simulink model "RoboBoatVU_2014_Dionysus"  (R2014a)
settings: Solver=FixedStepDiscrete  StartTime=0.0  StopTime=inf  FixedStep=.1  RelTol=1e-3
undefined symbols (not defined in the file): Com1, Com2, Com3, Com4, DiscIntNeverNeededParam, RGB24, standard
libraries: visiontextngfix x66, simulink x53, xpcseriallib x15, dspmtrx3 x14, slrtlib x3, speedgoatlib_IO102 x3, visionstatistics x2, dspstat3 x2, dspindex x2, xpcvideousblib x2, xpcvideoutillib x2, speedgoatlib x1
(part 1 of 7)
settings Model: BufferReuse=off  Creator=wildcat  LastModifiedBy=wildcat
settings SolverCC: EnableConcurrentExecution=on
settings DataIOCC: SignalLoggingSaveFormat=ModelDataLogs
settings OptimizationCC: BlockReduction=off  OptimizeBlockIOStorage=off  BufferReuse=off  GlobalBufferReuse=off  ExpressionFolding=off  LocalBlockOutputs=off
settings DebuggingCC: UnderspecifiedInitializationDetection=Classic  StateNameClashWarn=warning
settings HardwareCC: ProdIntDivRoundTo=Zero  ProdEndianess=LittleEndian  ProdHWDeviceType=Generic->32-bit x86 compatible
settings RTWCC: SystemTargetFile=slrt.tlc  TemplateMakefile=slrt_default_tmf  Description=Simulink Real-Time  ProcessScript=slrt_make_rtw_hook  RTWCompilerOptimization=On
settings SimulinkRealTimeCC: GeneratePreprocessorConditionals=Disable all  EnableShiftOperators=on

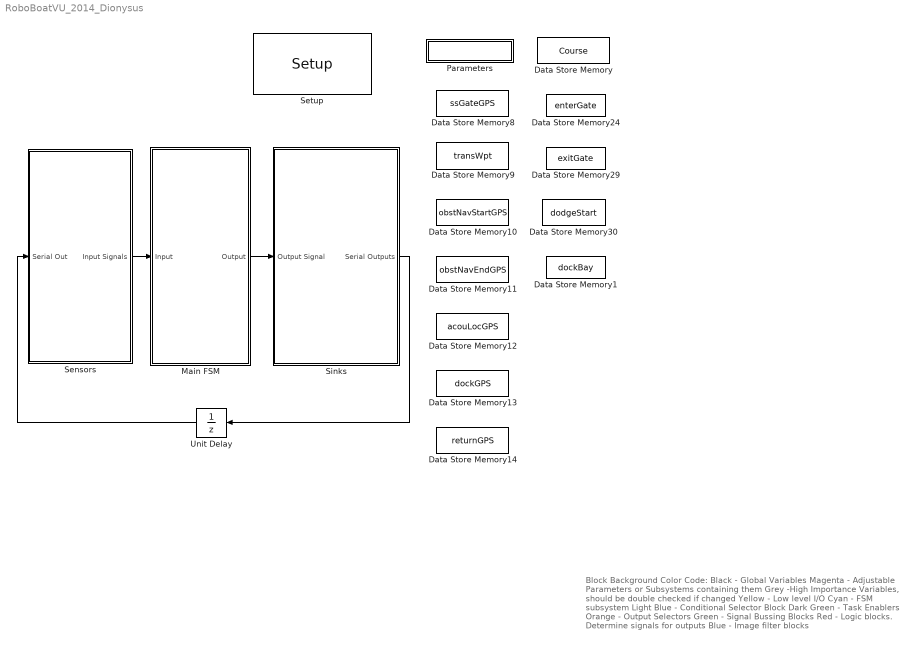
== system RoboBoatVU_2014_Dionysus ==
  note: Block Background Color Code:
      | Black - Global Variables
      | Magenta - Adjustable Parameters or Subsystems containing them
      | Grey -High Importance Variables, should be double checked if changed
      | Yellow - Low level I/O
      | Cyan - FSM subsystem
      | Light Blue - Conditional Selector Block
      | Dark Green - Task Enablers
      | Orange - Output Selectors
      | Green - Signal Bussing Blocks
      | Red - Logic blocks. Determine signals for outputs
      | Blue - Image filter blocks
  Data Store Memory : DataStoreMemory  DataStoreName=Course  ReadBeforeWriteMsg=warning  WriteAfterWriteMsg=warning  WriteAfterReadMsg=warning
  Data Store Memory1 : DataStoreMemory  DataStoreName=dockBay  ReadBeforeWriteMsg=warning  WriteAfterWriteMsg=warning  WriteAfterReadMsg=warning
  Data Store Memory10 : DataStoreMemory  DataStoreName=obstNavStartGPS  ReadBeforeWriteMsg=warning  WriteAfterWriteMsg=warning  WriteAfterReadMsg=warning  InitialValue=zeros(1,2)
  Data Store Memory11 : DataStoreMemory  DataStoreName=obstNavEndGPS  ReadBeforeWriteMsg=warning  WriteAfterWriteMsg=warning  WriteAfterReadMsg=warning  InitialValue=zeros(1,2)
  Data Store Memory12 : DataStoreMemory  DataStoreName=acouLocGPS  ReadBeforeWriteMsg=warning  WriteAfterWriteMsg=warning  WriteAfterReadMsg=warning  InitialValue=zeros(1,2)
  Data Store Memory13 : DataStoreMemory  DataStoreName=dockGPS  ReadBeforeWriteMsg=warning  WriteAfterWriteMsg=warning  WriteAfterReadMsg=warning  InitialValue=zeros(1,2)
  Data Store Memory14 : DataStoreMemory  DataStoreName=returnGPS  ReadBeforeWriteMsg=warning  WriteAfterWriteMsg=warning  WriteAfterReadMsg=warning  InitialValue=zeros(1,2)
  Data Store Memory24 : DataStoreMemory  DataStoreName=enterGate  ReadBeforeWriteMsg=warning  WriteAfterWriteMsg=warning  WriteAfterReadMsg=warning
  Data Store Memory29 : DataStoreMemory  DataStoreName=exitGate  ReadBeforeWriteMsg=warning  WriteAfterWriteMsg=warning  WriteAfterReadMsg=warning
  Data Store Memory30 : DataStoreMemory  DataStoreName=dodgeStart  ReadBeforeWriteMsg=warning  WriteAfterWriteMsg=warning  WriteAfterReadMsg=warning
  Data Store Memory8 : DataStoreMemory  DataStoreName=ssGateGPS  ReadBeforeWriteMsg=warning  WriteAfterWriteMsg=warning  WriteAfterReadMsg=warning  InitialValue=zeros(1,2)
  Data Store Memory9 : DataStoreMemory  DataStoreName=transWpt  ReadBeforeWriteMsg=warning  WriteAfterWriteMsg=warning  WriteAfterReadMsg=warning  InitialValue=zeros(1,2)
  Main FSM : Subsystem
  Parameters : Subsystem
  Sensors : Subsystem
  Setup : speedgoatlib_IO102/Setup  group=Digital output setup  id=1  range=+-5V  cal=off  pciSlot=-1  adChannelMode=Multiple-channel (enter number of channels below)  adChannel=16  adCoupling=Differential  daChannel=[1,2,3,4]  daReset=[1]  daInitValue=[0]  diChannel=[1,2,3,4,5,6,7,8]  doChannel=[1,2,3,4,5,6,7,8]  doReset=[1]  doInitValue=[0]
  Sinks : Subsystem
  Unit Delay : UnitDelay  SampleTime=-1
  wires:
  Main FSM/1(Output) -> Sinks/1(Output Signal)
  Sensors/1(Input Signals) -> Main FSM/1(Input)
  Sinks/1(Serial Outputs) -> Unit Delay/1
  Unit Delay/1 -> Sensors/1(Serial Out)

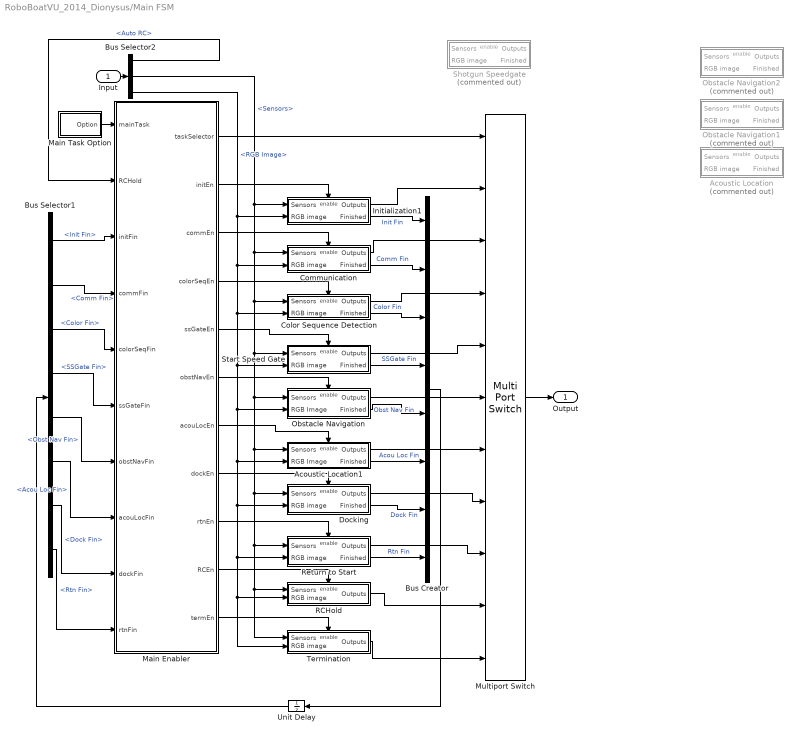
== system RoboBoatVU_2014_Dionysus/Main FSM ==
  Input : Inport
  Acoustic Location : Subsystem  Commented=on  TreatAsAtomicUnit=on
  Acoustic Location1 : Subsystem  TreatAsAtomicUnit=on
  Bus Creator : BusCreator  Inputs=8
  Bus Selector1 : BusSelector  OutputSignals=Init Fin,Comm Fin,Color Fin,SSGate Fin,Obst Nav Fin,Acou Loc Fin,Dock Fin,Rtn Fin
  Bus Selector2 : BusSelector  OutputSignals=Sensors.Digital In.Auto RC,Sensors,RGB Image
  Color Sequence Detection : Subsystem  TreatAsAtomicUnit=on
  Communication : Subsystem
  Docking : Subsystem  TreatAsAtomicUnit=on
  Initialization1 : Subsystem
  Main Enabler : MATLAB Function  TreatAsAtomicUnit=on
  Main Task Option : Subsystem
  Multiport Switch : MultiPortSwitch  Inputs=10
  Obstacle Navigation : Subsystem  TreatAsAtomicUnit=on
  Obstacle Navigation1 : Subsystem  Commented=on  TreatAsAtomicUnit=on
  Obstacle Navigation2 : Subsystem  Commented=on  TreatAsAtomicUnit=on
  RCHold : Subsystem
  Return to Start : Subsystem  TreatAsAtomicUnit=on
  Shotgun Speedgate : Subsystem  Commented=on  TreatAsAtomicUnit=on
  Start Speed Gate : Subsystem  TreatAsAtomicUnit=on
  Termination : Subsystem  TreatAsAtomicUnit=on
  Unit Delay : UnitDelay  SampleTime=-1
  Output : Outport
  wires:
  Bus Creator/1 -> Unit Delay/1
  Initialization1/1(Outputs) -> Multiport Switch/2
  Multiport Switch/1 -> Output/1
  Main Task Option/1(Option) -> Main Enabler/1(mainTask)
  Main Enabler/1(taskSelector) -> Multiport Switch/1
  Initialization1/2(Finished) -> Bus Creator/1  "Init Fin"
  Unit Delay/1 -> Bus Selector1/1
  Input/1 -> Bus Selector2/1
  Bus Selector2/1 -> Main Enabler/2(RCHold)  "<Auto RC>"
  Main Enabler/2(initEn) -> Initialization1/Enable
  Termination/1(Outputs) -> Multiport Switch/11
  RCHold/1(Outputs) -> Multiport Switch/10
  Main Enabler/10(RCEn) -> RCHold/Enable
  Main Enabler/11(termEn) -> Termination/Enable
  Bus Selector2/2 -> Communication/1(Sensors), Color Sequence Detection/1(Sensors), Start Speed Gate/1(Sensors), Obstacle Navigation/1(Sensors), Docking/1(Sensors), Return to Start/1(Sensors), RCHold/1(Sensors), Termination/1(Sensors), Acoustic Location1/1(Sensors), Initialization1/1(Sensors)  "<Sensors>"
  Bus Selector2/3 -> Communication/2(RGB image), Color Sequence Detection/2(RGB image), Start Speed Gate/2(RGB image), Obstacle Navigation/2(RGB Image), Docking/2(RGB image), Return to Start/2(RGB image), Termination/2(RGB image), RCHold/2(RGB image), Acoustic Location1/2(RGB Image), Initialization1/2(RGB image)  "<RGB Image>"
  Color Sequence Detection/2(Finished) -> Bus Creator/3  "Color Fin"
  Start Speed Gate/2(Finished) -> Bus Creator/4  "SSGate Fin"
  Obstacle Navigation/2(Finished) -> Bus Creator/5  "Obst Nav Fin"
  Acoustic Location1/2(Finished) -> Bus Creator/6  "Acou Loc Fin"
  Docking/2(Finished) -> Bus Creator/7  "Dock Fin"
  Return to Start/2(Finished) -> Bus Creator/8  "Rtn Fin"
  Return to Start/1(Outputs) -> Multiport Switch/9
  Docking/1(Outputs) -> Multiport Switch/8
  Acoustic Location1/1(Outputs) -> Multiport Switch/7
  Obstacle Navigation/1(Outputs) -> Multiport Switch/6
  Start Speed Gate/1(Outputs) -> Multiport Switch/5
  Color Sequence Detection/1(Outputs) -> Multiport Switch/4
  Main Enabler/4(colorSeqEn) -> Color Sequence Detection/Enable
  Main Enabler/5(ssGateEn) -> Start Speed Gate/Enable
  Main Enabler/6(obstNavEn) -> Obstacle Navigation/Enable
  Main Enabler/7(acouLocEn) -> Acoustic Location1/Enable
  Main Enabler/8(dockEn) -> Docking/Enable
  Main Enabler/9(rtnEn) -> Return to Start/Enable
  Bus Selector1/7 -> Main Enabler/9(dockFin)  "<Dock Fin>"
  Bus Selector1/1 -> Main Enabler/3(initFin)  "<Init Fin>"
  Bus Selector1/5 -> Main Enabler/7(obstNavFin)  "<Obst Nav Fin>"
  Bus Selector1/6 -> Main Enabler/8(acouLocFin)  "<Acou Loc Fin>"
  Bus Selector1/3 -> Main Enabler/5(colorSeqFin)  "<Color Fin>"
  Bus Selector1/4 -> Main Enabler/6(ssGateFin)  "<SSGate Fin>"
  Bus Selector1/8 -> Main Enabler/10(rtnFin)  "<Rtn Fin>"
  Main Enabler/3(commEn) -> Communication/Enable
  Communication/2(Finished) -> Bus Creator/2  "Comm Fin"
  Communication/1(Outputs) -> Multiport Switch/3
  Bus Selector1/2 -> Main Enabler/4(commFin)  "<Comm Fin>"

== system RoboBoatVU_2014_Dionysus/Parameters ==
  note: Course options are:
      | A, B and
      | otherwise (for testing,
      |  must be one character)
  CourseName : Constant  Value=uint8('B')  VectorParams1D=off
  GPS Points : Subsystem
  Write : DataStoreWrite  DataStoreName=Course
  wires:
  CourseName/1 -> Write/1

== system RoboBoatVU_2014_Dionysus/Sensors ==
  Serial Out : Inport
  Bus Creator : BusCreator  Inputs=2
  Bus Creator1 : BusCreator  Inputs=2
  Digital In : Subsystem
  Serial In : Subsystem
  Video In : Subsystem
  Input Signals : Outport
  wires:
  Serial In/1(Serial In) -> Bus Creator/1
  Digital In/1(Digital In) -> Bus Creator/2
  Video In/1(RGB image) -> Bus Creator1/2
  Bus Creator/1 -> Bus Creator1/1  "Sensors"
  Bus Creator1/1 -> Input Signals/1
  Serial Out/1 -> Serial In/1(Serial Out)

== system RoboBoatVU_2014_Dionysus/Sinks ==
  Output Signal : Inport
  Bus Selector : BusSelector  OutputSignals=Sensors.Serial In.Compass.Heading,Outputs.Control Signals,Outputs.Annotated Image,Outputs.Serial Outputs
  Image Transmission : Subsystem
  actuators : Subsystem
  data log : Subsystem  Commented=on
  Serial Outputs : Outport
  wires:
  Bus Selector/2 -> actuators/2(Control Signals)  "<Control Signals>"
  Bus Selector/3 -> Image Transmission/1(RGB Image)  "<Annotated Image>"
  Bus Selector/1 -> actuators/1(Compass Heading)  "<Heading>"
  Output Signal/1 -> data log/1(Output signal), Bus Selector/1
  Bus Selector/4 -> Serial Outputs/1  "<Serial Outputs>"

== system RoboBoatVU_2014_Dionysus/Main FSM/Acoustic Location ==
  note: Acoustic Location
  Sensors : Inport
  RGB image : Inport  Port=2
  Enable : EnablePort  ShowOutputPort=on
  Annotate Task : visiontextngfix/Insert Text  inputType=Obsolete  theText='Acoustic Location...'  getTextLocFrom=Specify via dialog  textLoc=[10 10]  getTextColorFrom=Specify via dialog  textColor=[0 0 255]  getTextIntensityFrom=Specify via dialog  textIntensity=0  getTextOpacityFrom=Specify via dialog  textOpacity=1.0  dummyVar2=0  dummyVar3=0  dummyVar4=0  imagePorts=One multidimensional signal  isInputTransposed=off  fontFace=LucidaSansRegular  dummyVar1=0  blockFontSize=12  antiAliased=on
  Bus Selector : BusSelector  OutputSignals=Serial In.Compass.Heading
  Compare To Constant : simulink/Logic and Bit Operations/Compare To Constant  relop=>=  const=10  OutDataTypeStr=boolean
  Constant : Constant  Value=0
  Data Type Conversion : DataTypeConversion  OutDataTypeStr=double
  Discrete-Time Integrator : DiscreteIntegrator  SampleTime=0.1  ICPrevOutput=DiscIntNeverNeededParam  ICPrevScaledInput=DiscIntNeverNeededParam
  Output Heirarchy : Subsystem
  Outputs : Outport
  Finished : Outport  Port=2
  wires:
  Sensors/1 -> Output Heirarchy/3(Sensors), Bus Selector/1  "Sensors"
  Bus Selector/1 -> Output Heirarchy/2(Desired Heading)  "<Heading>"
  RGB image/1 -> Annotate Task/1
  Annotate Task/1 -> Output Heirarchy/1(Annotated Image)
  Output Heirarchy/1(Outputs) -> Outputs/1
  Compare To Constant/1 -> Data Type Conversion/1
  Enable/1 -> Discrete-Time Integrator/1
  Discrete-Time Integrator/1 -> Compare To Constant/1
  Constant/1 -> Output Heirarchy/4(Request Number)
  Data Type Conversion/1 -> Finished/1

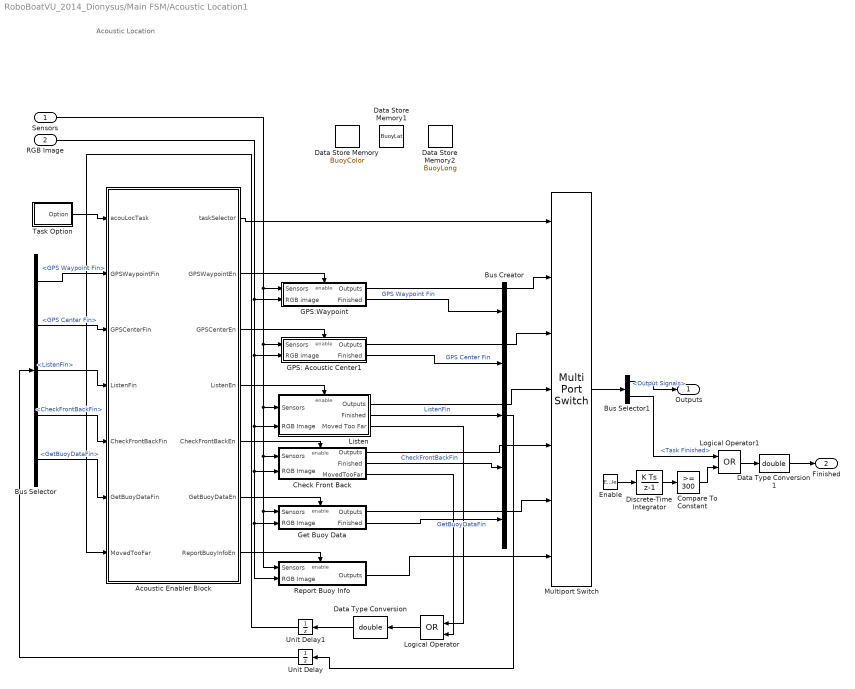
== system RoboBoatVU_2014_Dionysus/Main FSM/Acoustic Location1 ==
  note: Acoustic Location
  Sensors : Inport
  RGB Image : Inport  Port=2
  Enable : EnablePort  ShowOutputPort=on
  Acoustic Enabler Block : MATLAB Function  TreatAsAtomicUnit=on
  Bus Creator : BusCreator  Inputs=5
  Bus Selector : BusSelector  OutputSignals=GPS Waypoint Fin,GPS Center Fin,ListenFin,CheckFrontBackFin,GetBuoyDataFin
  Bus Selector1 : BusSelector  OutputSignals=Output Signals,Task Finished
  Check Front Back : Subsystem  TreatAsAtomicUnit=on
  Compare To Constant : simulink/Logic and Bit Operations/Compare To Constant  relop=>=  const=300  OutDataTypeStr=boolean
  Data Store Memory : DataStoreMemory  DataStoreName=BuoyColor  ReadBeforeWriteMsg=warning  WriteAfterWriteMsg=warning  WriteAfterReadMsg=warning
  Data Store Memory1 : DataStoreMemory  DataStoreName=BuoyLat  ReadBeforeWriteMsg=warning  WriteAfterWriteMsg=warning  WriteAfterReadMsg=warning
  Data Store Memory2 : DataStoreMemory  DataStoreName=BuoyLong  ReadBeforeWriteMsg=warning  WriteAfterWriteMsg=warning  WriteAfterReadMsg=warning
  Data Type Conversion : DataTypeConversion  OutDataTypeStr=double
  Data Type Conversion1 : DataTypeConversion  OutDataTypeStr=double
  Discrete-Time Integrator : DiscreteIntegrator  SampleTime=0.1  ICPrevOutput=DiscIntNeverNeededParam  ICPrevScaledInput=DiscIntNeverNeededParam
  GPS: Acoustic Center1 : Subsystem  TreatAsAtomicUnit=on
  GPS:Waypoint : Subsystem  TreatAsAtomicUnit=on
  Get Buoy Data : Subsystem  TreatAsAtomicUnit=on
  Listen : Subsystem  TreatAsAtomicUnit=on
  Logical Operator : Logic  Operator=OR  IconShape=distinctive  AllPortsSameDT=off  OutDataTypeStr=boolean
  Logical Operator1 : Logic  Operator=OR  AllPortsSameDT=off  OutDataTypeStr=boolean
  Multiport Switch : MultiPortSwitch  Inputs=6
  Report Buoy Info : Subsystem  TreatAsAtomicUnit=on
  Task Option : Subsystem
  Unit Delay : UnitDelay  SampleTime=-1
  Unit Delay1 : UnitDelay  SampleTime=-1
  Outputs : Outport
  Finished : Outport  Port=2
  wires:
  Sensors/1 -> GPS:Waypoint/1(Sensors), GPS: Acoustic Center1/1(Sensors), Report Buoy Info/1(Sensors), Get Buoy Data/1(Sensors), Check Front Back/1(Sensors), Listen/1(Sensors)
  RGB Image/1 -> GPS:Waypoint/2(RGB image), GPS: Acoustic Center1/2(RGB image), Report Buoy Info/2(RGB Image), Get Buoy Data/2(RGB Image), Check Front Back/2(RGB Image), Listen/2(RGB Image)
  Acoustic Enabler Block/1(taskSelector) -> Multiport Switch/1
  Acoustic Enabler Block/3(GPSCenterEn) -> GPS: Acoustic Center1/Enable
  Acoustic Enabler Block/4(ListenEn) -> Listen/Enable
  Acoustic Enabler Block/5(CheckFrontBackEn) -> Check Front Back/Enable
  Acoustic Enabler Block/7(ReportBuoyInfoEn) -> Report Buoy Info/Enable
  Listen/1(Outputs) -> Multiport Switch/4
  Check Front Back/1(Outputs) -> Multiport Switch/5
  Report Buoy Info/1(Outputs) -> Multiport Switch/7
  Listen/2(Finished) -> Bus Creator/3  "ListenFin"
  Check Front Back/2(Finished) -> Bus Creator/4  "CheckFrontBackFin"
  Unit Delay/1 -> Bus Selector/1
  Bus Selector/2 -> Acoustic Enabler Block/3(GPSCenterFin)  "<GPS Center Fin>"
  Multiport Switch/1 -> Bus Selector1/1
  GPS: Acoustic Center1/1(Outputs) -> Multiport Switch/3
  GPS: Acoustic Center1/2(Finished) -> Bus Creator/2  "GPS Center Fin"
  Bus Creator/1 -> Unit Delay/1
  Get Buoy Data/1(Outputs) -> Multiport Switch/6
  Get Buoy Data/2(Finished) -> Bus Creator/5  "GetBuoyDataFin"
  Bus Selector/5 -> Acoustic Enabler Block/6(GetBuoyDataFin)  "<GetBuoyDataFin>"
  Bus Selector/3 -> Acoustic Enabler Block/4(ListenFin)  "<ListenFin>"
  Bus Selector/4 -> Acoustic Enabler Block/5(CheckFrontBackFin)  "<CheckFrontBackFin>"
  Acoustic Enabler Block/6(GetBuoyDataEn) -> Get Buoy Data/Enable
  Task Option/1(Option) -> Acoustic Enabler Block/1(acouLocTask)
  Listen/3(Moved Too Far) -> Logical Operator/1
  Unit Delay1/1 -> Acoustic Enabler Block/7(MovedTooFar)
  Check Front Back/3(MovedTooFar) -> Logical Operator/2
  Logical Operator/1 -> Data Type Conversion/1
  Data Type Conversion/1 -> Unit Delay1/1
  Acoustic Enabler Block/2(GPSWaypointEn) -> GPS:Waypoint/Enable
  GPS:Waypoint/1(Outputs) -> Multiport Switch/2
  GPS:Waypoint/2(Finished) -> Bus Creator/1  "GPS Waypoint Fin"
  Bus Selector1/1 -> Outputs/1  "<Output Signals>"
  Bus Selector/1 -> Acoustic Enabler Block/2(GPSWaypointFin)  "<GPS Waypoint Fin>"
  Enable/1 -> Discrete-Time Integrator/1
  Discrete-Time Integrator/1 -> Compare To Constant/1
  Logical Operator1/1 -> Data Type Conversion1/1
  Bus Selector1/2 -> Logical Operator1/1  "<Task Finished>"
  Compare To Constant/1 -> Logical Operator1/2
  Data Type Conversion1/1 -> Finished/1

== system RoboBoatVU_2014_Dionysus/Main FSM/Color Sequence Detection ==
  note: Color Sequence Detection
  Sensors : Inport
  RGB image : Inport  Port=2
  Enable : EnablePort
  Main Enabler : MATLAB Function  TreatAsAtomicUnit=on
  Main Selector : MultiPortSwitch  Inputs=2
  Output Reassign : Subsystem
  Report : Subsystem  TreatAsAtomicUnit=on
  Request : Subsystem  TreatAsAtomicUnit=on
  Unit Delay : UnitDelay  SampleTime=-1
  Outputs : Outport
  Finished : Outport  Port=2
  wires:
  Main Enabler/2(RequestEn) -> Request/Enable
  Sensors/1 -> Request/1(Sensors), Report/1(Sensors)
  RGB image/1 -> Request/2(RGB image), Report/2(RGB image)
  Request/1(Outputs) -> Main Selector/2
  Report/1(Outputs) -> Main Selector/3
  Request/2(Finished) -> Unit Delay/1
  Unit Delay/1 -> Main Enabler/1(RequestFin)
  Main Enabler/1(taskSelector) -> Main Selector/1
  Main Enabler/3(ReportEn) -> Report/Enable
  Main Selector/1 -> Output Reassign/1(Outputs in)
  Output Reassign/1(Outputs) -> Outputs/1
  Output Reassign/2(Finished) -> Finished/1

== system RoboBoatVU_2014_Dionysus/Main FSM/Communication ==
  Sensors : Inport
  RGB image : Inport  Port=2
  Enable : EnablePort
  Docking Bay Comm : Subsystem  TreatAsAtomicUnit=on
  Main Enabler : MATLAB Function  TreatAsAtomicUnit=on
  Main Selector : MultiPortSwitch  Inputs=2
  Obst Gate Comm : Subsystem  TreatAsAtomicUnit=on
  Output Reassign : Subsystem
  Unit Delay : UnitDelay  SampleTime=-1
  Outputs : Outport
  Finished : Outport  Port=2
  wires:
  Main Enabler/2(ObstCommEn) -> Obst Gate Comm/Enable
  Sensors/1 -> Docking Bay Comm/1(Sensors), Obst Gate Comm/1(Sensors)
  RGB image/1 -> Docking Bay Comm/2(RGB image), Obst Gate Comm/2(RGB image)
  Obst Gate Comm/1(Outputs) -> Main Selector/2
  Docking Bay Comm/1(Outputs) -> Main Selector/3
  Obst Gate Comm/2(Finished) -> Unit Delay/1
  Unit Delay/1 -> Main Enabler/1(ObstCommFin)
  Main Enabler/1(taskSelector) -> Main Selector/1
  Main Enabler/3(DockingCommEn) -> Docking Bay Comm/Enable
  Main Selector/1 -> Output Reassign/1(Outputs in)
  Output Reassign/1(Outputs) -> Outputs/1
  Output Reassign/2(Finished) -> Finished/1

== system RoboBoatVU_2014_Dionysus/Main FSM/Docking ==
  note: Docking
  Sensors : Inport
  RGB image : Inport  Port=2
  Enable : EnablePort  ShowOutputPort=on
  Annotate Task : visiontextngfix/Insert Text  inputType=Obsolete  theText='Docking...'  getTextLocFrom=Specify via dialog  textLoc=[10 10]  getTextColorFrom=Specify via dialog  textColor=[0 0 255]  getTextIntensityFrom=Specify via dialog  textIntensity=0  getTextOpacityFrom=Specify via dialog  textOpacity=1.0  dummyVar2=0  dummyVar3=0  dummyVar4=0  imagePorts=One multidimensional signal  isInputTransposed=off  fontFace=LucidaSansRegular  dummyVar1=0  blockFontSize=12  antiAliased=on
  Annotate Task1 : visiontextngfix/Insert Text  inputType=Obsolete  theText='Symbol: %f'  getTextLocFrom=Specify via dialog  textLoc=[10 20]  getTextColorFrom=Specify via dialog  textColor=[0 0 255]  getTextIntensityFrom=Specify via dialog  textIntensity=0  getTextOpacityFrom=Specify via dialog  textOpacity=1.0  dummyVar2=0  dummyVar3=0  dummyVar4=0  imagePorts=One multidimensional signal  isInputTransposed=off  fontFace=LucidaSansRegular  dummyVar1=0  blockFontSize=12  antiAliased=on
  Bus Selector : BusSelector  OutputSignals=Serial In.Comms.Dat1,Serial In.Compass.Heading
  Compare To Constant : simulink/Logic and Bit Operations/Compare To Constant  relop=>=  const=5  OutDataTypeStr=boolean
  Constant : Constant  Value=2
  Data Type Conversion : DataTypeConversion  OutDataTypeStr=double
  Discrete-Time Integrator : DiscreteIntegrator  SampleTime=0.1  ICPrevOutput=DiscIntNeverNeededParam  ICPrevScaledInput=DiscIntNeverNeededParam
  Output Heirarchy : Subsystem
  Outputs : Outport
  Finished : Outport  Port=2
  wires:
  Sensors/1 -> Bus Selector/1, Output Heirarchy/3(Sensors)  "Sensors"
  Bus Selector/2 -> Output Heirarchy/2(Desired Heading)  "<Heading>"
  RGB image/1 -> Annotate Task/1
  Output Heirarchy/1(Outputs) -> Outputs/1
  Compare To Constant/1 -> Data Type Conversion/1
  Enable/1 -> Discrete-Time Integrator/1
  Discrete-Time Integrator/1 -> Compare To Constant/1
  Constant/1 -> Output Heirarchy/4(Request Number)
  Annotate Task/1 -> Annotate Task1/1
  Bus Selector/1 -> Annotate Task1/2  "<Dat1>"
  Annotate Task1/1 -> Output Heirarchy/1(Annotated Image)
  Data Type Conversion/1 -> Finished/1

== system RoboBoatVU_2014_Dionysus/Main FSM/Initialization1 ==
  Sensors : Inport
  RGB image : Inport  Port=2
  Enable : EnablePort  ShowOutputPort=on
  Annotate Task : visiontextngfix/Insert Text  inputType=Obsolete  theText='Initializing...'  getTextLocFrom=Specify via dialog  textLoc=[10 10]  getTextColorFrom=Specify via dialog  textColor=[0 0 255]  getTextIntensityFrom=Specify via dialog  textIntensity=0  getTextOpacityFrom=Specify via dialog  textOpacity=1.0  dummyVar2=0  dummyVar3=0  dummyVar4=0  imagePorts=One multidimensional signal  isInputTransposed=off  fontFace=LucidaSansRegular  dummyVar1=0  blockFontSize=12  antiAliased=on
  Bus Selector : BusSelector  OutputSignals=Serial In.Compass.Heading
  Compare To Constant : simulink/Logic and Bit Operations/Compare To Constant  relop=>=  const=5  OutDataTypeStr=boolean
  Constant : Constant  Value=0
  Data Type Conversion : DataTypeConversion  OutDataTypeStr=double
  Discrete-Time Integrator : DiscreteIntegrator  SampleTime=0.1  ICPrevOutput=DiscIntNeverNeededParam  ICPrevScaledInput=DiscIntNeverNeededParam
  Output Heirarchy : Subsystem
  Outputs : Outport
  Finished : Outport  Port=2
  wires:
  Sensors/1 -> Bus Selector/1, Output Heirarchy/3(Sensors)  "Sensors"
  Bus Selector/1 -> Output Heirarchy/2(Desired Heading)  "<Heading>"
  RGB image/1 -> Annotate Task/1
  Annotate Task/1 -> Output Heirarchy/1(Annotated Image)
  Output Heirarchy/1(Outputs) -> Outputs/1
  Compare To Constant/1 -> Data Type Conversion/1
  Enable/1 -> Discrete-Time Integrator/1
  Discrete-Time Integrator/1 -> Compare To Constant/1
  Constant/1 -> Output Heirarchy/4(Request Number)
  Data Type Conversion/1 -> Finished/1

== system RoboBoatVU_2014_Dionysus/Main FSM/Main Task Option ==
  note: Main Task Options
  Message Composer : MATLAB Function  TreatAsAtomicUnit=on
  Test Comms Option : Constant  Value=uint8('All')  SampleTime=0.1
  Option : Outport
  wires:
  Test Comms Option/1 -> Message Composer/1(taskStrInit)
  Message Composer/1(taskStrAdj) -> Option/1

== system RoboBoatVU_2014_Dionysus/Main FSM/Obstacle Navigation ==
  note: Distance threshold changed from 2m to 3m
  note: Variables to test:
      | 1. RPM values for GPS approach and dodge subroutine
      | 2. Angle threshold for ignoring obstacle
  note: Places to change RPM value
      | Dodge/Nav Logic: 2 places
      | GPS: Bee Line/Approach/Output Heirarchy1: 1 place
  Sensors : Inport
  RGB Image : Inport  Port=2
  Enable : EnablePort  ShowOutputPort=on
  Compare To Constant1 : simulink/Logic and Bit Operations/Compare To Constant  relop=>=  const=180  OutDataTypeStr=boolean
  Data Store Read : DataStoreRead  DataStoreName=dodgeStart  SampleTime=0.1
  Data Type Conversion1 : DataTypeConversion  OutDataTypeStr=double
  Discrete-Time Integrator : DiscreteIntegrator  SampleTime=0.1  ICPrevOutput=DiscIntNeverNeededParam  ICPrevScaledInput=DiscIntNeverNeededParam
  Dodge : Subsystem  TreatAsAtomicUnit=on
  GPS: Bee Line : Subsystem  TreatAsAtomicUnit=on
  Logical Operator : Logic  Operator=OR  AllPortsSameDT=off  OutDataTypeStr=boolean
  Multiport Switch : MultiPortSwitch  Inputs=2
  Obstacle Navigation Enabler : MATLAB Function  TreatAsAtomicUnit=on
  Output Reassign : Subsystem
  Unit Delay : UnitDelay  SampleTime=-1
  Outputs : Outport
  Finished : Outport  Port=2
  wires:
  Obstacle Navigation Enabler/3(GPSEn) -> GPS: Bee Line/Enable
  Sensors/1 -> GPS: Bee Line/1(Sensors), Dodge/1(Sensors)
  RGB Image/1 -> GPS: Bee Line/2(RGB image), Dodge/2(RGB image)
  Obstacle Navigation Enabler/2(dodgeEn) -> Dodge/Enable
  Dodge/1(Outputs) -> Multiport Switch/2
  GPS: Bee Line/1(Outputs) -> Multiport Switch/3
  Obstacle Navigation Enabler/1(taskSelector) -> Multiport Switch/1
  Dodge/2(Dodge Incomplete) -> Unit Delay/1  "Dodge Incomplete"
  Data Store Read/1 -> Obstacle Navigation Enabler/2(dodgeStart)
  Unit Delay/1 -> Obstacle Navigation Enabler/1(dodgeIncomplete)
  Multiport Switch/1 -> Output Reassign/1(Outputs in)
  Output Reassign/1(Outputs) -> Outputs/1
  Output Reassign/2(Finished) -> Logical Operator/2
  Discrete-Time Integrator/1 -> Compare To Constant1/1
  Compare To Constant1/1 -> Logical Operator/1
  Enable/1 -> Discrete-Time Integrator/1
  Logical Operator/1 -> Data Type Conversion1/1
  Data Type Conversion1/1 -> Finished/1

== system RoboBoatVU_2014_Dionysus/Main FSM/Obstacle Navigation1 ==
  Sensors : Inport
  RGB image : Inport  Port=2
  Enable : EnablePort
  Bus Creator1 : BusCreator
  Bus Selector1 : BusSelector  OutputSignals=GPS Fin,Comm Fin,Enter Fin,Nav Fin
  Communication : Subsystem  TreatAsAtomicUnit=on
  Enter Gate : Subsystem  TreatAsAtomicUnit=on
  Exit Gate : Subsystem  TreatAsAtomicUnit=on
  GPS: Center : Subsystem  TreatAsAtomicUnit=on
  MATLAB Function1 : MATLAB Function  TreatAsAtomicUnit=on
  Multiport Switch1 : MultiPortSwitch  Inputs=5
  Obstacle Navigation : Subsystem  TreatAsAtomicUnit=on
  Output Reassign : Subsystem
  Task Option1 : Subsystem
  Unit Delay1 : UnitDelay  SampleTime=-1
  Outputs : Outport
  Finished : Outport  Port=2
  wires:
  Task Option1/1(Option) -> MATLAB Function1/1(taskMode)
  MATLAB Function1/2(startGPSEn) -> GPS: Center/Enable
  GPS: Center/1(Outputs) -> Multiport Switch1/2
  MATLAB Function1/1(taskSelector) -> Multiport Switch1/1
  MATLAB Function1/3(commEn) -> Communication/Enable
  MATLAB Function1/6(exitGateEn) -> Exit Gate/Enable
  MATLAB Function1/5(obstNavEn) -> Obstacle Navigation/Enable
  MATLAB Function1/4(enterGateEn) -> Enter Gate/Enable
  GPS: Center/2(Finished) -> Bus Creator1/1  "GPS Fin"
  Communication/2(Finished) -> Bus Creator1/2  "Comm Fin"
  Enter Gate/2(Finished) -> Bus Creator1/3  "Enter Fin"
  Obstacle Navigation/2(Finished) -> Bus Creator1/4  "Nav Fin"
  Obstacle Navigation/1(Outputs) -> Multiport Switch1/5
  Enter Gate/1(Outputs) -> Multiport Switch1/4
  Communication/1(Outputs) -> Multiport Switch1/3
  Bus Creator1/1 -> Unit Delay1/1
  Unit Delay1/1 -> Bus Selector1/1
  Bus Selector1/1 -> MATLAB Function1/2(startGPSFin)  "<GPS Fin>"
  Bus Selector1/2 -> MATLAB Function1/3(commFin)  "<Comm Fin>"
  Bus Selector1/3 -> MATLAB Function1/4(enterGateFin)  "<Enter Fin>"
  Bus Selector1/4 -> MATLAB Function1/5(obstNavFin)  "<Nav Fin>"
  Exit Gate/1(Outputs) -> Multiport Switch1/6
  Sensors/1 -> GPS: Center/1(Sensors), Communication/1(Sensors), Enter Gate/1(Sensors), Exit Gate/1(Sensors), Obstacle Navigation/1(Sensors)
  RGB image/1 -> GPS: Center/2(RGB image), Communication/2(RGB Image), Enter Gate/2(RGB Image), Exit Gate/2(RGB Image), Obstacle Navigation/2(RGB Image)
  Multiport Switch1/1 -> Output Reassign/1(Outputs in)
  Output Reassign/1(Outputs) -> Outputs/1
  Output Reassign/2(Finished) -> Finished/1

== system RoboBoatVU_2014_Dionysus/Main FSM/Obstacle Navigation2 ==
  note: Obstacle Navigation
  Sensors : Inport
  RGB image : Inport  Port=2
  Enable : EnablePort  ShowOutputPort=on
  Annotate Task : visiontextngfix/Insert Text  inputType=Obsolete  theText='Obstacle Nav...'  getTextLocFrom=Specify via dialog  textLoc=[10 10]  getTextColorFrom=Specify via dialog  textColor=[0 0 255]  getTextIntensityFrom=Specify via dialog  textIntensity=0  getTextOpacityFrom=Specify via dialog  textOpacity=1.0  dummyVar2=0  dummyVar3=0  dummyVar4=0  imagePorts=One multidimensional signal  isInputTransposed=off  fontFace=LucidaSansRegular  dummyVar1=0  blockFontSize=12  antiAliased=on
  Annotate Task1 : visiontextngfix/Insert Text  inputType=Obsolete  theText='Enter Gate: %f'  getTextLocFrom=Specify via dialog  textLoc=[10 20]  getTextColorFrom=Specify via dialog  textColor=[0 0 255]  getTextIntensityFrom=Specify via dialog  textIntensity=0  getTextOpacityFrom=Specify via dialog  textOpacity=1.0  dummyVar2=0  dummyVar3=0  dummyVar4=0  imagePorts=One multidimensional signal  isInputTransposed=off  fontFace=LucidaSansRegular  dummyVar1=0  blockFontSize=12  antiAliased=on
  Annotate Task2 : visiontextngfix/Insert Text  inputType=Obsolete  theText='Exit Gate: %f'  getTextLocFrom=Specify via dialog  textLoc=[10 30]  getTextColorFrom=Specify via dialog  textColor=[0 0 255]  getTextIntensityFrom=Specify via dialog  textIntensity=0  getTextOpacityFrom=Specify via dialog  textOpacity=1.0  dummyVar2=0  dummyVar3=0  dummyVar4=0  imagePorts=One multidimensional signal  isInputTransposed=off  fontFace=LucidaSansRegular  dummyVar1=0  blockFontSize=12  antiAliased=on
  Bus Selector : BusSelector  OutputSignals=Serial In.Comms.Dat1,Serial In.Comms.Dat2,Serial In.Compass.Heading,Serial In.Comms.CP
  Compare To Constant : simulink/Logic and Bit Operations/Compare To Constant  relop=>=  const=60  OutDataTypeStr=boolean
  Constant : Constant
  Data Type Conversion : DataTypeConversion  OutDataTypeStr=double
  Discrete-Time Integrator : DiscreteIntegrator  SampleTime=0.1  ICPrevOutput=DiscIntNeverNeededParam  ICPrevScaledInput=DiscIntNeverNeededParam
  Logical Operator : Logic  Operator=OR  AllPortsSameDT=off  OutDataTypeStr=boolean
  MATLAB Function : MATLAB Function  TreatAsAtomicUnit=on
  Output Heirarchy : Subsystem
  Outputs : Outport
  Finished : Outport  Port=2
  wires:
  Sensors/1 -> Bus Selector/1, Output Heirarchy/3(Sensors)  "Sensors"
  Bus Selector/3 -> Output Heirarchy/2(Desired Heading)  "<Heading>"
  RGB image/1 -> Annotate Task/1
  Output Heirarchy/1(Outputs) -> Outputs/1
  Enable/1 -> Discrete-Time Integrator/1
  Discrete-Time Integrator/1 -> Compare To Constant/1
  Annotate Task/1 -> Annotate Task1/1
  Bus Selector/1 -> Annotate Task1/2  "<Dat1>"
  Annotate Task1/1 -> Annotate Task2/1
  Bus Selector/2 -> Annotate Task2/2  "<Dat2>"
  Annotate Task2/1 -> Output Heirarchy/1(Annotated Image)
  Data Type Conversion/1 -> Finished/1
  MATLAB Function/2(Finished) -> Logical Operator/1
  Compare To Constant/1 -> Logical Operator/2
  Logical Operator/1 -> Data Type Conversion/1
  MATLAB Function/1(requestNumOut) -> Output Heirarchy/4(Request Number)
  Constant/1 -> MATLAB Function/2(requestNumIn)
  Bus Selector/4 -> MATLAB Function/1(CP)  "<CP>"

== system RoboBoatVU_2014_Dionysus/Main FSM/RCHold ==
  Sensors : Inport
  RGB image : Inport  Port=2
  Enable : EnablePort
  Annotate Task : visiontextngfix/Insert Text  inputType=Obsolete  theText='RC Hold'  getTextLocFrom=Specify via dialog  textLoc=[10 10]  getTextColorFrom=Specify via dialog  textColor=[0 0 255]  getTextIntensityFrom=Specify via dialog  textIntensity=0  getTextOpacityFrom=Specify via dialog  textOpacity=1.0  dummyVar2=0  dummyVar3=0  dummyVar4=0  imagePorts=One multidimensional signal  isInputTransposed=off  fontFace=LucidaSansRegular  dummyVar1=0  blockFontSize=12  antiAliased=on
  Bus Selector : BusSelector  OutputSignals=Serial In.Compass.Heading
  Output Heirarchy : Subsystem
  Outputs : Outport
  wires:
  Sensors/1 -> Output Heirarchy/3(Sensors), Bus Selector/1  "Sensors"
  Bus Selector/1 -> Output Heirarchy/1(Desired Heading)  "<Heading>"
  RGB image/1 -> Annotate Task/1
  Annotate Task/1 -> Output Heirarchy/2(Annotated Image)
  Output Heirarchy/1(Outputs) -> Outputs/1

== system RoboBoatVU_2014_Dionysus/Main FSM/Return to Start ==
  note: Return to Start
  Sensors : Inport
  RGB image : Inport  Port=2
  Enable : EnablePort  ShowOutputPort=on
  Annotate Task : visiontextngfix/Insert Text  inputType=Obsolete  theText='Return...'  getTextLocFrom=Specify via dialog  textLoc=[10 10]  getTextColorFrom=Specify via dialog  textColor=[0 0 255]  getTextIntensityFrom=Specify via dialog  textIntensity=0  getTextOpacityFrom=Specify via dialog  textOpacity=1.0  dummyVar2=0  dummyVar3=0  dummyVar4=0  imagePorts=One multidimensional signal  isInputTransposed=off  fontFace=LucidaSansRegular  dummyVar1=0  blockFontSize=12  antiAliased=on
  Bus Selector : BusSelector  OutputSignals=Serial In.Compass.Heading
  Compare To Constant : simulink/Logic and Bit Operations/Compare To Constant  relop=>=  const=5  OutDataTypeStr=boolean
  Data Type Conversion : DataTypeConversion  OutDataTypeStr=double
  Discrete-Time Integrator : DiscreteIntegrator  SampleTime=0.1  ICPrevOutput=DiscIntNeverNeededParam  ICPrevScaledInput=DiscIntNeverNeededParam
  Output Heirarchy : Subsystem
  Outputs : Outport
  Finished : Outport  Port=2
  wires:
  Sensors/1 -> Bus Selector/1, Output Heirarchy/3(Sensors)  "Sensors"
  Bus Selector/1 -> Output Heirarchy/2(Desired Heading)  "<Heading>"
  RGB image/1 -> Annotate Task/1
  Annotate Task/1 -> Output Heirarchy/1(Annotated Image)
  Output Heirarchy/1(Outputs) -> Outputs/1
  Compare To Constant/1 -> Data Type Conversion/1
  Enable/1 -> Discrete-Time Integrator/1
  Discrete-Time Integrator/1 -> Compare To Constant/1
  Data Type Conversion/1 -> Finished/1

== system RoboBoatVU_2014_Dionysus/Main FSM/Shotgun Speedgate ==
  note: Start Speed Gate
  Sensors : Inport
  RGB image : Inport  Port=2
  Enable : EnablePort  ShowOutputPort=on
  Bus Selector : BusSelector  OutputSignals=Serial In.Compass.Heading
  Compare To Constant : simulink/Logic and Bit Operations/Compare To Constant  relop=>=  const=60  OutDataTypeStr=boolean
  Constant : Constant  Value=4000
  Data Type Conversion : DataTypeConversion  OutDataTypeStr=double
  Insert Text : visiontextngfix/Insert Text  inputType=Obsolete  theText='SSGate Shotgun'  getTextLocFrom=Specify via dialog  textLoc=[1 1]  getTextColorFrom=Specify via dialog  textColor=[0 0 0]  getTextIntensityFrom=Specify via dialog  textIntensity=0  getTextOpacityFrom=Specify via dialog  textOpacity=1.0  dummyVar2=0  dummyVar3=0  dummyVar4=0  imagePorts=One multidimensional signal  isInputTransposed=off  fontFace=LucidaSansRegular  dummyVar1=0  blockFontSize=12  antiAliased=on
  MATLAB Function : MATLAB Function  TreatAsAtomicUnit=on
  MATLAB Function1 : MATLAB Function  TreatAsAtomicUnit=on
  Output Heirarchy : Subsystem
  "Scope " : slrtlib/Displays and Logging/Scope   scopeno=1  scopetype=File  autostart=on  viewmode=Graphical redraw  formatstr='%15.6f'  grid=on  ylimits=[0,0]  nosamples=300  noprepostsamples=0  interleave=1  triggermode=FreeRun  triggersignal=1  trigsignalfromport=off  triggerlevel=0.0  triggerslope=Either  triggerscope=1  triggersample=0  filename=ssgate.dat  mode=Lazy  writesize=512  autorestart=off  dynamicfilemode=off  maxwritefilesize=512*1024^2
  Timer : DiscreteIntegrator  SampleTime=-1  ICPrevOutput=DiscIntNeverNeededParam  ICPrevScaledInput=DiscIntNeverNeededParam
  Outputs : Outport
  Finished : Outport  Port=2
  wires:
  RGB image/1 -> Insert Text/1
  Sensors/1 -> Output Heirarchy/1(Sensors), Bus Selector/1  "Sensors"
  Enable/1 -> Timer/1
  Timer/1 -> Compare To Constant/1
  Output Heirarchy/1(Outputs) -> Outputs/1
  Data Type Conversion/1 -> Finished/1
  Compare To Constant/1 -> Data Type Conversion/1
  Constant/1 -> Output Heirarchy/3(RPM)
  Bus Selector/1 -> MATLAB Function1/2(Heading), MATLAB Function/1(Heading)  "<Heading>"
  MATLAB Function/1(LockedHeading) -> MATLAB Function1/1(desiredHeading), Output Heirarchy/4(Desired Heading)
  Insert Text/1 -> Output Heirarchy/2(Annotated Image)
  MATLAB Function1/1(out) -> "Scope "/1

== system RoboBoatVU_2014_Dionysus/Main FSM/Start Speed Gate ==
  note: Start Speed Gate
  Sensors : Inport
  RGB image : Inport  Port=2
  Enable : EnablePort  ShowOutputPort=on
  Buoy Decisions : Subsystem
  Bus Selector : BusSelector  OutputSignals=Serial In.GPS.latitude,Serial In.GPS.longitude
  Constant : Constant  Value=120
  Nav Finished : MATLAB Function  TreatAsAtomicUnit=on
  Output Heirarchy : Subsystem
  Read : DataStoreRead  DataStoreName=obstNavStartGPS  SampleTime=0.1
  Start Speed Gate Detection : Subsystem
  Timer : DiscreteIntegrator  SampleTime=-1  ICPrevOutput=DiscIntNeverNeededParam  ICPrevScaledInput=DiscIntNeverNeededParam
  Outputs : Outport
  Finished : Outport  Port=2
  wires:
  RGB image/1 -> Buoy Decisions/2(RGB image), Start Speed Gate Detection/1(RGB)
  Sensors/1 -> Output Heirarchy/1(Sensors), Bus Selector/1, Buoy Decisions/1(Sensors)  "Sensors"
  Start Speed Gate Detection/1(Red + Green) -> Buoy Decisions/3(Red + Green)
  Enable/1 -> Timer/1
  Timer/1 -> Nav Finished/1(Timer), Buoy Decisions/4(Timer)
  Read/1 -> Nav Finished/3(DesiredGPS)
  Bus Selector/2 -> Nav Finished/5(GPSLong)  "<longitude>"
  Bus Selector/1 -> Nav Finished/4(GPSLat)  "<latitude>"
  Buoy Decisions/1(Annotated Image) -> Output Heirarchy/2(Annotated Image)
  Output Heirarchy/1(Outputs) -> Outputs/1
  Constant/1 -> Nav Finished/2(Timeout)
  Buoy Decisions/2(RPM) -> Output Heirarchy/3(RPM)
  Buoy Decisions/3(Desired Heading) -> Output Heirarchy/4(Desired Heading)
  Nav Finished/1(Finished) -> Finished/1

== system RoboBoatVU_2014_Dionysus/Main FSM/Termination ==
  Sensors : Inport
  RGB image : Inport  Port=2
  Enable : EnablePort
  Annotate Task : visiontextngfix/Insert Text  inputType=Obsolete  theText='Terminating...'  getTextLocFrom=Specify via dialog  textLoc=[10 10]  getTextColorFrom=Specify via dialog  textColor=[0 0 255]  getTextIntensityFrom=Specify via dialog  textIntensity=0  getTextOpacityFrom=Specify via dialog  textOpacity=1.0  dummyVar2=0  dummyVar3=0  dummyVar4=0  imagePorts=One multidimensional signal  isInputTransposed=off  fontFace=LucidaSansRegular  dummyVar1=0  blockFontSize=12  antiAliased=on
  Bus Selector : BusSelector  OutputSignals=Serial In.Compass.Heading
  Output Heirarchy : Subsystem
  Outputs : Outport
  wires:
  RGB image/1 -> Annotate Task/1
  Annotate Task/1 -> Output Heirarchy/1(Annotated Image)  "Annotated Image"
  Output Heirarchy/1(Outputs) -> Outputs/1
  Sensors/1 -> Bus Selector/1, Output Heirarchy/3(Sensors)  "Sensors"
  Bus Selector/1 -> Output Heirarchy/2(Desired Heading)  "<Heading>"

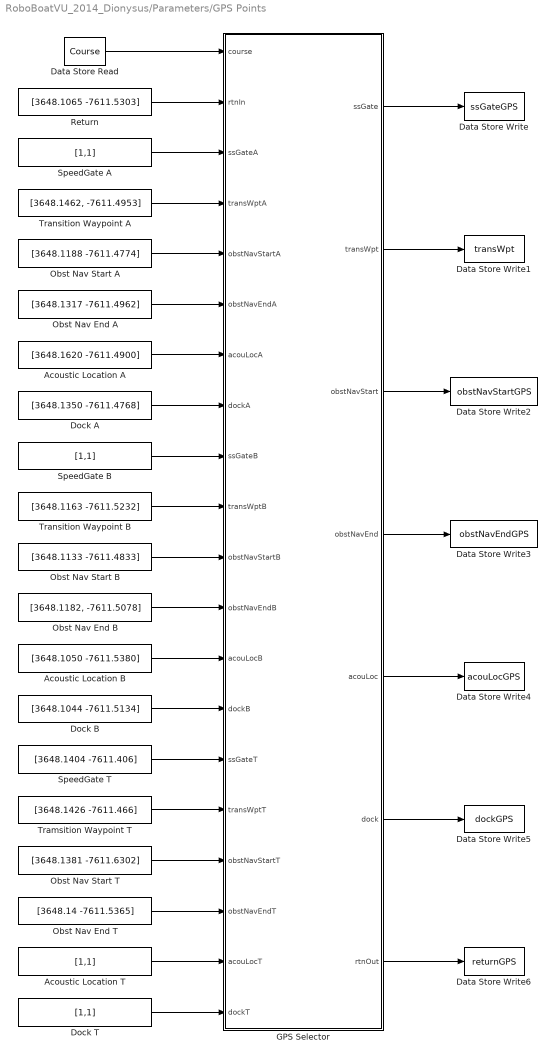
== system RoboBoatVU_2014_Dionysus/Parameters/GPS Points ==
  Acoustic Location A : Constant  Value=[3648.1620 -7611.4900]  SampleTime=0.1
  Acoustic Location B : Constant  Value=[3648.1050 -7611.5380]  SampleTime=0.1
  Acoustic Location T : Constant  Value=[1,1]  SampleTime=0.1
  Data Store Read : DataStoreRead  DialogController=Simulink.DDGSource  DataStoreName=Course  SampleTime=0.1
  Data Store Write : DataStoreWrite  DialogController=Simulink.DDGSource  DataStoreName=ssGateGPS
  Data Store Write1 : DataStoreWrite  DataStoreName=transWpt
  Data Store Write2 : DataStoreWrite  DataStoreName=obstNavStartGPS
  Data Store Write3 : DataStoreWrite  DataStoreName=obstNavEndGPS
  Data Store Write4 : DataStoreWrite  DataStoreName=acouLocGPS
  Data Store Write5 : DataStoreWrite  DataStoreName=dockGPS
  Data Store Write6 : DataStoreWrite  DataStoreName=returnGPS
  Dock A : Constant  Value=[3648.1350 -7611.4768]  SampleTime=0.1
  Dock B : Constant  Value=[3648.1044 -7611.5134]  SampleTime=0.1
  Dock T : Constant  Value=[1,1]  SampleTime=0.1
  GPS Selector : MATLAB Function  TreatAsAtomicUnit=on
  Obst Nav End A : Constant  Value=[3648.1317 -7611.4962]  SampleTime=0.1
  Obst Nav End B : Constant  Value=[3648.1182, -7611.5078]  SampleTime=0.1
  Obst Nav End T : Constant  Value=[3648.14 -7611.5365]  SampleTime=0.1
  Obst Nav Start A : Constant  Value=[3648.1188 -7611.4774]  SampleTime=0.1
  Obst Nav Start B : Constant  Value=[3648.1133 -7611.4833]  SampleTime=0.1
  Obst Nav Start T : Constant  Value=[3648.1381 -7611.6302]  SampleTime=0.1
  Return : Constant  Value=[3648.1065 -7611.5303]  SampleTime=0.1
  SpeedGate A : Constant  Value=[1,1]  SampleTime=0.1
  SpeedGate B : Constant  Value=[1,1]  SampleTime=0.1
  SpeedGate T : Constant  Value=[3648.1404 -7611.406]  SampleTime=0.1
  Tramsition Waypoint T : Constant  Value=[3648.1426 -7611.466]  SampleTime=0.1
  Transition Waypoint A : Constant  Value=[3648.1462, -7611.4953]  SampleTime=0.1
  Transition Waypoint B : Constant  Value=[3648.1163 -7611.5232]  SampleTime=0.1
  wires:
  Data Store Read/1 -> GPS Selector/1(course)
  Return/1 -> GPS Selector/2(rtnIn)
  SpeedGate A/1 -> GPS Selector/3(ssGateA)
  Transition Waypoint A/1 -> GPS Selector/4(transWptA)
  Obst Nav Start A/1 -> GPS Selector/5(obstNavStartA)
  Obst Nav End A/1 -> GPS Selector/6(obstNavEndA)
  SpeedGate T/1 -> GPS Selector/15(ssGateT)
  Acoustic Location T/1 -> GPS Selector/19(acouLocT)
  Tramsition Waypoint T/1 -> GPS Selector/16(transWptT)
  Dock A/1 -> GPS Selector/8(dockA)
  Dock T/1 -> GPS Selector/20(dockT)
  Obst Nav End T/1 -> GPS Selector/18(obstNavEndT)
  Obst Nav Start T/1 -> GPS Selector/17(obstNavStartT)
  Obst Nav Start B/1 -> GPS Selector/11(obstNavStartB)
  Obst Nav End B/1 -> GPS Selector/12(obstNavEndB)
  Acoustic Location A/1 -> GPS Selector/7(acouLocA)
  Acoustic Location B/1 -> GPS Selector/13(acouLocB)
  Dock B/1 -> GPS Selector/14(dockB)
  SpeedGate B/1 -> GPS Selector/9(ssGateB)
  Transition Waypoint B/1 -> GPS Selector/10(transWptB)
  GPS Selector/1(ssGate) -> Data Store Write/1
  GPS Selector/2(transWpt) -> Data Store Write1/1
  GPS Selector/3(obstNavStart) -> Data Store Write2/1
  GPS Selector/4(obstNavEnd) -> Data Store Write3/1
  GPS Selector/5(acouLoc) -> Data Store Write4/1
  GPS Selector/6(dock) -> Data Store Write5/1
  GPS Selector/7(rtnOut) -> Data Store Write6/1

== system RoboBoatVU_2014_Dionysus/Sensors/Digital In ==
  Bus Creator : BusCreator  Inputs=1
  Digital input : speedgoatlib_IO102/Digital input  id=1  channels=[1,2,3,4,5,6,7,8]  ts=0.1  pciSlot=-1
  Terminator{1,17..22} (7 alike) : Terminator
  Digital In : Outport
  wires:
  Bus Creator/1 -> Digital In/1  "Digital In"
  Digital input/8 -> Bus Creator/1  "Auto RC"
  Digital input/2 -> Terminator17/1
  Digital input/3 -> Terminator18/1
  Digital input/4 -> Terminator19/1
  Digital input/5 -> Terminator20/1
  Digital input/6 -> Terminator21/1
  Digital input/7 -> Terminator22/1
  Digital input/1 -> Terminator1/1

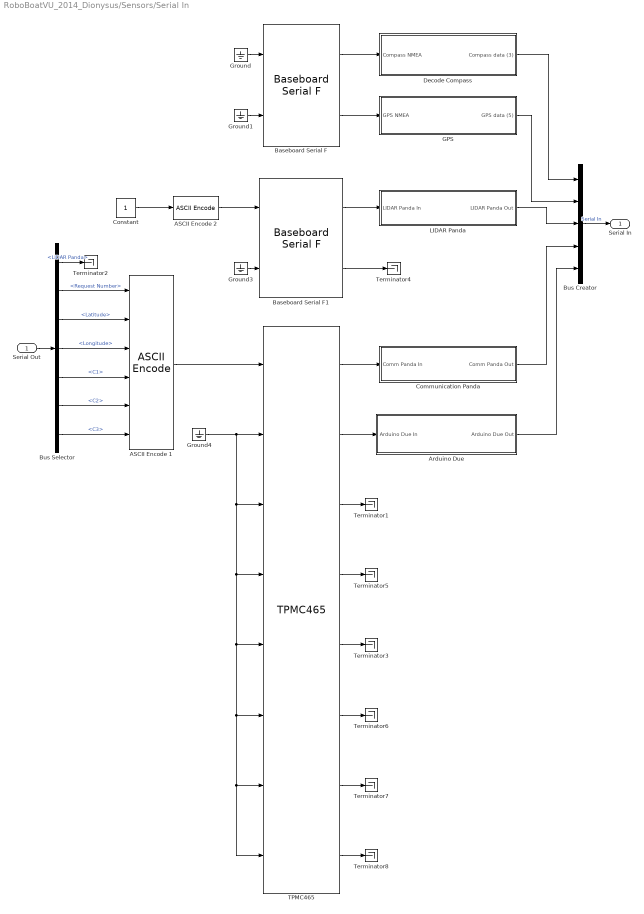
== system RoboBoatVU_2014_Dionysus/Sensors/Serial In ==
  Serial Out : Inport
  " GPS" : Subsystem
  ASCII Encode 1 : xpcseriallib/ASCII Encode   format="{\"SGR\":%d,\"Lat\":%f,\"Long\":%f,\"C1\":%d,\"C2\":%d,\"C3\":%d} \\r\\n"  nvars=6  maxlength=128  vartypes={ 'double' }
  ASCII Encode 2 : xpcseriallib/ASCII Encode   format=SGTask:%d \r\n  nvars=1  maxlength=128  vartypes={ 'double' }
  Arduino Due : Subsystem
  Baseboard Serial F : xpcseriallib/Mainboard/Baseboard Serial F  group=Basic Setup  port=2  irqnum=4  saddr1=0x3f8  saddr2=0x3e8  config=Com1/Com3  baud1=19200  parity1=None  ndata1=8  nstop1=1  fifomode1=64 deep  rlevel1=half full  automode1=on  xmtfifosize1=1024  xmtdatatype1=8 bit uint null terminated  rcvfifosize1=1024  baud2=19200  parity2=None  ndata2=8  nstop2=1  fifomode2=64 deep  rlevel2=half full  automode2=on  xmtfifosize2=1024  xmtdatatype2=8 bit uint null terminated  rcvfifosize2=1024
  Baseboard Serial F1 : xpcseriallib/Mainboard/Baseboard Serial F  group=Basic Setup  port=1  irqnum=4  saddr1=0x3f8  saddr2=0x3e8  config=Com2/Com4  baud1=115200  parity1=None  ndata1=8  nstop1=1  fifomode1=64 deep  rlevel1=half full  automode1=on  xmtfifosize1=1024  xmtdatatype1=8 bit uint null terminated  rcvfifosize1=1024  baud2=115200  parity2=None  ndata2=8  nstop2=1  fifomode2=64 deep  rlevel2=half full  automode2=on  xmtfifosize2=1024  xmtdatatype2=8 bit uint null terminated  rcvfifosize2=1024
  Bus Creator : BusCreator  Inputs=5
  Bus Selector : BusSelector  OutputSignals=LIDAR Panda,Comms Panda.Request Number,Comms Panda.Latitude,Comms Panda.Longitude,Comms Panda.C1,Comms Panda.C2,Comms Panda.C3
  Communication Panda : Subsystem
  Constant : Constant
  Decode Compass : Subsystem
  Ground{,1,3..4} (4 alike) : Ground
  LIDAR Panda : Subsystem
  TPMC465 : speedgoatlib/IO504/TPMC465  group=Basic Setup  port=2  irqnum=9  slot=-1  transceiver1=RS232 (max 921.6kb/s)  standard1=on  baud1=115200  bauddivisor1=1  sampling1=16x (standard)  prescale1=off  parity1=Even  ndata1=7  nstop1=1  rlevel1=half full (32)  hwmode1=none  swmode1=none  xonchar1=17  xoffchar1=19  rs485auto1=off  rs485delay1=0  xmtfifosize1=1024  xmtdatatype1=8 bit uint null terminated  rcvfifosize1=1024  transceiver2=RS232 (max 921.6kb/s)  standard2=on  baud2=115200  bauddivisor2=1  sampling2=16x (standard)  prescale2=off  parity2=None  ndata2=8  nstop2=1  rlevel2=half full (32)  hwmode2=none  swmode2=none  xonchar2=17  xoffchar2=19  rs485auto2=off  rs485delay2=0  xmtfifosize2=1024  xmtdatatype2=8 bit uint null terminated  rcvfifosize2=1024  transceiver3=RS232 (max 921.6kb/s)  standard3=on  baud3=115200  bauddivisor3=1  sampling3=16x (standard)  prescale3=off  parity3=None  ndata3=8  nstop3=1  rlevel3=half full (32)  hwmode3=none  swmode3=none  xonchar3=17  xoffchar3=19  rs485auto3=off  rs485delay3=0  xmtfifosize3=1024  xmtdatatype3=8 bit uint null terminated  rcvfifosize3=1024  transceiver4=RS232 (max 921.6kb/s)  standard4=on  baud4=115200  bauddivisor4=1  sampling4=16x (standard)  prescale4=off  parity4=None  ndata4=8  nstop4=1  rlevel4=half full (32)  hwmode4=none  swmode4=none  xonchar4=17  xoffchar4=19  rs485auto4=off  rs485delay4=0  xmtfifosize4=1024  xmtdatatype4=8 bit uint null terminated  rcvfifosize4=1024  transceiver5=RS232 (max 921.6kb/s)  standard5=on  baud5=115200  bauddivisor5=1  sampling5=16x (standard)  prescale5=off  parity5=None  ndata5=8  nstop5=1  rlevel5=1  hwmode5=none  swmode5=none  xonchar5=17  xoffchar5=19  rs485auto5=off  rs485delay5=0  xmtfifosize5=1024  xmtdatatype5=8 bit uint null terminated  rcvfifosize5=1024  transceiver6=RS232 (max 921.6kb/s)  standard6=on  baud6=115200  bauddivisor6=1  sampling6=16x (standard)  prescale6=off  parity6=None  ndata6=8  nstop6=1  rlevel6=1  hwmode6=none  swmode6=none  xonchar6=17  xoffchar6=19  rs485auto6=off  rs485delay6=0  xmtfifosize6=1024  xmtdatatype6=8 bit uint null terminated  rcvfifosize6=1024  transceiver7=RS232 (max 921.6kb/s)  standard7=on  baud7=115200  bauddivisor7=1  sampling7=16x (standard)  prescale7=off  parity7=None  ndata7=8  nstop7=1  rlevel7=1  hwmode7=none  swmode7=none  xonchar7=17  xoffchar7=19  rs485auto7=off  rs485delay7=0  xmtfifosize7=1024  xmtdatatype7=8 bit uint null terminated  rcvfifosize7=1024  transceiver8=RS232 (max 921.6kb/s)  standard8=on  baud8=115200  bauddivisor8=1  sampling8=16x (standard)  prescale8=off  parity8=None  ndata8=8  nstop8=1  rlevel8=1  hwmode8=none  swmode8=none  xonchar8=17  xoffchar8=19  rs485auto8=off  rs485delay8=0  xmtfifosize8=1024  xmtdatatype8=8 bit uint null terminated  rcvfifosize8=1024
  Terminator{1..8} (8 alike) : Terminator
  Serial In : Outport
  wires:
  Decode Compass/1(Compass data (3)) -> Bus Creator/1
  " GPS"/1(GPS data (5)) -> Bus Creator/2
  Bus Creator/1 -> Serial In/1  "Serial In"
  Ground4/1 -> TPMC465/3, TPMC465/6, TPMC465/8, TPMC465/7, TPMC465/5, TPMC465/4, TPMC465/2
  TPMC465/6 -> Terminator6/1
  TPMC465/7 -> Terminator7/1
  TPMC465/8 -> Terminator8/1
  TPMC465/5 -> Terminator3/1
  Communication Panda/1(Comm Panda Out) -> Bus Creator/4
  Ground/1 -> Baseboard Serial F/1
  Ground1/1 -> Baseboard Serial F/2
  Baseboard Serial F/1 -> Decode Compass/1(Compass NMEA)
  Ground3/1 -> Baseboard Serial F1/2
  Arduino Due/1(Arduino Due Out) -> Bus Creator/5
  TPMC465/4 -> Terminator5/1
  TPMC465/1 -> Communication Panda/1(Comm Panda In)
  TPMC465/2 -> Arduino Due/1(Arduino Due In)
  Baseboard Serial F1/2 -> Terminator4/1
  Baseboard Serial F/2 -> " GPS"/1(GPS NMEA)
  TPMC465/3 -> Terminator1/1
  Baseboard Serial F1/1 -> LIDAR Panda/1(LIDAR Panda In)
  LIDAR Panda/1(LIDAR Panda Out) -> Bus Creator/3
  ASCII Encode 1/1 -> TPMC465/1
  Serial Out/1 -> Bus Selector/1
  Bus Selector/7 -> ASCII Encode 1/6  "<C3>"
  Bus Selector/6 -> ASCII Encode 1/5  "<C2>"
  Bus Selector/2 -> ASCII Encode 1/1  "<Request Number>"
  Bus Selector/3 -> ASCII Encode 1/2  "<Latitude>"
  Bus Selector/5 -> ASCII Encode 1/4  "<C1>"
  Bus Selector/4 -> ASCII Encode 1/3  "<Longitude>"
  ASCII Encode 2/1 -> Baseboard Serial F1/1
  Bus Selector/1 -> Terminator2/1  "<LIDAR Panda>"
  Constant/1 -> ASCII Encode 2/1

== system RoboBoatVU_2014_Dionysus/Sensors/Video In ==
  From USB Video Device : xpcvideousblib/From USB Video Device  sconf=<Select a configuration>  paddr=-1  iwidth=640  iheight=480  fint=1/10  ffmt=Uncompressed  cfmt=RGB24 (8:8:8)  isig=One multidimensional signal  trigger=off  status=off  updateBlock=1
  USB Video Device List : xpcvideousblib/USB Video Device List  usb_search=on  ShowInLibBrowser=0
  RGB image : Outport
  wires:
  From USB Video Device/1 -> RGB image/1  "RGB Image"

== system RoboBoatVU_2014_Dionysus/Sinks/Image Transmission ==
  note: Image Transmission
  RGB Image : Inport
  Image Transmit : xpcvideoutillib/Image Transmit  ipAddress=255.255.255.255  ipPort=25000  localPort=-1  vblLen=on  maxpacket=40*1024  sampletime=-1
  Jpeg Compression1 : xpcvideoutillib/Jpeg Compression  quality=40  cspace=RGB  isig=One multidimensional signal  maxsize=640*480  length=on
  Rate Transition : RateTransition  OutPortSampleTime=1
  wires:
  Jpeg Compression1/1 -> Image Transmit/1
  Jpeg Compression1/2 -> Image Transmit/2
  Rate Transition/1 -> Jpeg Compression1/1
  RGB Image/1 -> Rate Transition/1

== system RoboBoatVU_2014_Dionysus/Sinks/actuators ==
  Compass Heading : Inport
  Control Signals : Inport  Port=2
  analog output : Subsystem
  wires:
  Control Signals/1 -> analog output/2(Control Signals)
  Compass Heading/1 -> analog output/1(Compass Heading)
